simulink model "Lab1_with_PID"  (R2014b)
settings: Solver=ode45  StartTime=0.0  StopTime=10.0  RelTol=1e-3
undefined symbols (not defined in the file): b, g, I, l, M, m
libraries: simulink x1
settings Model: Creator=nrjbasu  LastModifiedBy=nrjbasu
settings DebuggingCC: AlgebraicLoopMsg=none

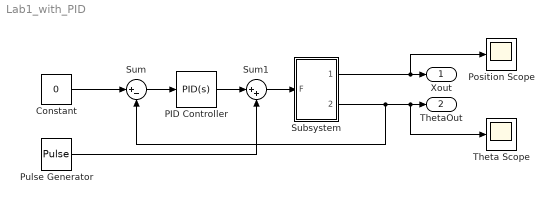
== system Lab1_with_PID ==
  Constant : Constant  Value=0
  PID Controller : simulink/Continuous/PID Controller  Controller=PID  TimeDomain=Continuous-time  SampleTime=-1  IntegratorMethod=Forward Euler  FilterMethod=Forward Euler  Form=Parallel  P=100  I=1  D=20  N=100  InitialConditionSource=internal  InitialConditionForIntegrator=0  InitialConditionForFilter=0  ExternalReset=none  LimitOutput=off  UpperSaturationLimit=inf  LowerSaturationLimit=-inf  LinearizeAsGain=on  AntiWindupMode=none  Kb=1  TrackingMode=off  Kt=1  PParamMin=[]  PParamMax=[]  IParamMin=[]  IParamMax=[]  DParamMin=[]  DParamMax=[]  NParamMin=[]  NParamMax=[]  KbParamMin=[]  KbParamMax=[]  KtParamMin=[]  KtParamMax=[]  POutMin=[]  POutMax=[]  IOutMin=[]  IOutMax=[]  DOutMin=[]  DOutMax=[]  NOutMin=[]  NOutMax=[]  KbOutMin=[]  KbOutMax=[]  KtOutMin=[]  KtOutMax=[]  IntegratorOutMin=[]  IntegratorOutMax=[]  FilterOutMin=[]  FilterOutMax=[]  SumOutMin=[]  SumOutMax=[]  SumI1OutMin=[]  SumI1OutMax=[]  SumI2OutMin=[]  SumI2OutMax=[]  SumI3OutMin=[]  SumI3OutMax=[]  SumDOutMin=[]  SumDOutMax=[]  SaturationOutMin=[]  SaturationOutMax=[]  IntegratorContinuousStateAttributes=''  IntegratorStateMustResolveToSignalObject=off  IntegratorRTWStateStorageClass=Auto  FilterContinuousStateAttributes=''  FilterStateMustResolveToSignalObject=off  FilterRTWStateStorageClass=Auto  DifferentiatorICPrevScaledInput=0  DifferentiatorOutMin=[]  DifferentiatorOutMax=[]  UseFilter=on
  Position Scope : Scope
      settings: TimeRange=10  YMin=-0.2  YMax=1
  Pulse Generator : DiscretePulseGenerator  PulseType=Time based  Amplitude=1000  Period=10  PulseWidth=.001
  Subsystem : Subsystem
  Sum : Sum  Inputs=|+-
  Sum1 : Sum  Inputs=|++
  Theta Scope : Scope
  Xout : Outport
  ThetaOut : Outport  Port=2
  wires:
  Subsystem/1(Xout) -> Position Scope/1, Xout/1
  Constant/1 -> Sum/1
  Sum/1 -> PID Controller/1
  PID Controller/1 -> Sum1/1
  Subsystem/2(Thetaout) -> Sum/2, Theta Scope/1, ThetaOut/1
  Pulse Generator/1 -> Sum1/2
  Sum1/1 -> Subsystem/1(F)

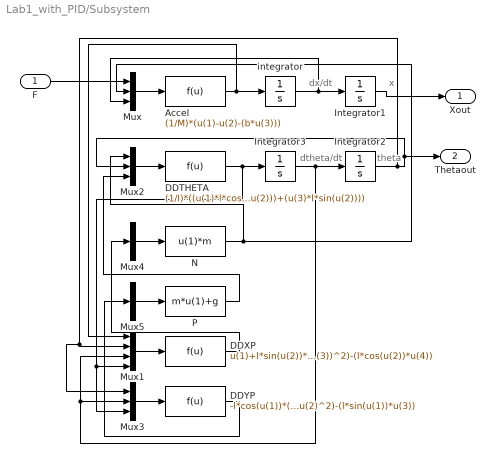
== system Lab1_with_PID/Subsystem ==
  note: x
  note: theta
  note: dtheta/dt
  note: dx/dt
  F : Inport
  Accel : Fcn  Expr=(1/M)*(u(1)-u(2)-(b*u(3)))
  DDTHETA : Fcn  Expr=(1/I)*((u(1)*l*cos(u(2)))+(u(3)*l*sin(u(2))))
  DDXP : Fcn  Expr=u(1)+l*sin(u(2))*((u(3))^2)-(l*cos(u(2))*u(4))
  DDYP : Fcn  Expr=-l*cos(u(1))*(u(2)^2)-(l*sin(u(1))*u(3))
  Integrator1 : Integrator
  Integrator2 : Integrator
  Integrator3 : Integrator
  Mux : Mux  Inputs=3
  Mux1 : Mux
  Mux2 : Mux  Inputs=3
  Mux3 : Mux  Inputs=3
  Mux4 : Mux  Inputs=1
  Mux5 : Mux  Inputs=1
  N : Fcn  Expr=u(1)*m
  P : Fcn  Expr=m*u(1)+g
  integrator : Integrator
  Xout : Outport
  Thetaout : Outport  Port=2
  wires:
  P/1 -> Mux2/3
  F/1 -> Mux/1
  N/1 -> Mux2/1, Mux/2
  Integrator1/1 -> Xout/1
  DDTHETA/1 -> Mux1/4, Mux3/3, Integrator3/1
  Accel/1 -> Mux1/1, integrator/1
  Integrator2/1 -> Mux3/1, Mux1/2, Thetaout/1, Mux2/2
  Integrator3/1 -> Mux3/2, Mux1/3, Integrator2/1
  Mux/1 -> Accel/1
  Mux3/1 -> DDYP/1
  Mux2/1 -> DDTHETA/1
  Mux1/1 -> DDXP/1
  integrator/1 -> Mux/3, Integrator1/1
  Mux4/1 -> N/1
  Mux5/1 -> P/1
  DDXP/1 -> Mux4/1
  DDYP/1 -> Mux5/1
